simulink model "bpsk_rx_coarse_sync"  (R2020a)
settings: Solver=VariableStepAuto  StartTime=0.0  StopTime=10.0  RelTol=1e-3
undefined symbols (not defined in the file): AXI4, designMultirateFIR, Lite, tx_data, xlfda_numerator
libraries: xbsIndex_r4 x68, hdlsllib x11, dspmlti4 x10, dspswit3 x4, dspsigops x2, commrandsrc3 x1, simulink x1
(part 2 of 2)

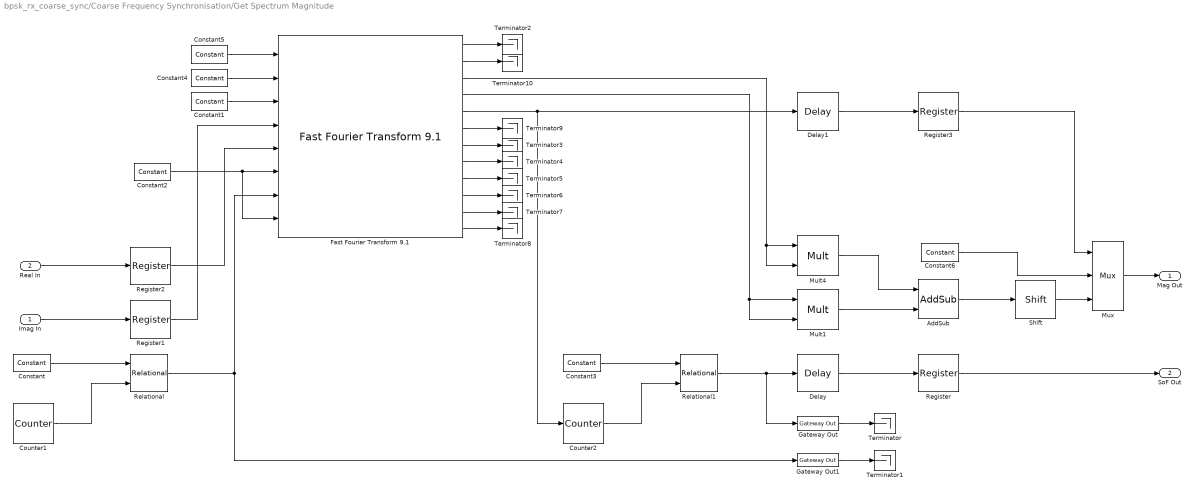
== system bpsk_rx_coarse_sync/Coarse Frequency Synchronisation/Get Spectrum Magnitude ==
  Imag In : Inport
  Real In : Inport  Port=2
  AddSub : xbsIndex_r4/AddSub  mode=Addition  use_carryin=off  use_carryout=off  en=off  latency=1  precision=Full  arith_type=Unsigned  n_bits=16  bin_pt=14  quantization=Truncate  overflow=Wrap  use_behavioral_HDL=off  hw_selection=Fabric  pipelined=off  dbl_ovrd=off  block_type=addsub
  Constant : xbsIndex_r4/Constant  const=1023  gui_display_data_type=Fixed-point  arith_type=Unsigned  n_bits=10  bin_pt=0  preci_type=Single  exp_width=8  frac_width=24  explicit_period=on  period=1/12.8e6  equ=P=C  opselect=C  inp2=PCIN>>17  opr=+  inp1=P  carry=CIN  dbl_ovrd=off  block_type=constant
  Constant1 : xbsIndex_r4/Constant  const=0  gui_display_data_type=Boolean  arith_type=Boolean  n_bits=16  bin_pt=14  preci_type=Single  exp_width=8  frac_width=24  explicit_period=on  period=1/12.8e6  equ=P=C  opselect=C  inp2=PCIN>>17  opr=+  inp1=P  carry=CIN  dbl_ovrd=off  block_type=constant
  Constant2 : xbsIndex_r4/Constant  const=1  gui_display_data_type=Boolean  arith_type=Boolean  n_bits=16  bin_pt=14  preci_type=Single  exp_width=8  frac_width=24  explicit_period=on  period=1/12.8e6  equ=P=C  opselect=C  inp2=PCIN>>17  opr=+  inp1=P  carry=CIN  dbl_ovrd=off  block_type=constant
  Constant3 : xbsIndex_r4/Constant  const=0  gui_display_data_type=Fixed-point  arith_type=Unsigned  n_bits=10  bin_pt=0  preci_type=Single  exp_width=8  frac_width=24  explicit_period=on  period=1/12.8e6  equ=P=C  opselect=C  inp2=PCIN>>17  opr=+  inp1=P  carry=CIN  dbl_ovrd=off  block_type=constant
  Constant4 : xbsIndex_r4/Constant  const=0  gui_display_data_type=Fixed-point  arith_type=Unsigned  n_bits=1  bin_pt=0  preci_type=Single  exp_width=8  frac_width=24  explicit_period=on  period=1/12.8e6  equ=P=C  opselect=C  inp2=PCIN>>17  opr=+  inp1=P  carry=CIN  dbl_ovrd=off  block_type=constant
  Constant5 : xbsIndex_r4/Constant  const=0  gui_display_data_type=Fixed-point  arith_type=Unsigned  n_bits=10  bin_pt=0  preci_type=Single  exp_width=8  frac_width=24  explicit_period=on  period=1/12.8e6  equ=P=C  opselect=C  inp2=PCIN>>17  opr=+  inp1=P  carry=CIN  dbl_ovrd=off  block_type=constant
  Constant6 : xbsIndex_r4/Constant  const=0  gui_display_data_type=Fixed-point  arith_type=Unsigned  n_bits=32  bin_pt=31  preci_type=Single  exp_width=8  frac_width=24  explicit_period=on  period=1/12.8e6  equ=P=C  opselect=C  inp2=PCIN>>17  opr=+  inp1=P  carry=CIN  dbl_ovrd=off  block_type=constant
  Counter1 : xbsIndex_r4/Counter  cnt_type=Count Limited  cnt_to=1023  operation=Up  start_count=0  cnt_by_val=1  arith_type=Unsigned  n_bits=10  bin_pt=0  load_pin=off  rst=off  en=off  explicit_period=on  period=1/12.8e6  use_behavioral_HDL=off  implementation=Fabric  dbl_ovrd=off  block_type=counter
  Counter2 : xbsIndex_r4/Counter  cnt_type=Count Limited  cnt_to=1023  operation=Up  start_count=0  cnt_by_val=1  arith_type=Unsigned  n_bits=10  bin_pt=0  load_pin=off  rst=off  en=on  explicit_period=on  period=1/12.8e6  use_behavioral_HDL=off  implementation=Fabric  dbl_ovrd=off  block_type=counter
  Delay : xbsIndex_r4/Delay  rst=off  infoeditControl=Selection of Reset will increase slice count due to use of real FFs and instead of SRLs  en=off  latency=3  reg_retiming=off  dbl_ovrd=off  block_type=delay
  Delay1 : xbsIndex_r4/Delay  rst=off  infoeditControl=Selection of Reset will increase slice count due to use of real FFs and instead of SRLs  en=off  latency=3  reg_retiming=off  dbl_ovrd=off  block_type=delay
  "Fast Fourier Transform 9.1 " : xbsIndex_r4/Fast Fourier Transform 9.1   transform_length=1024  target_clock_frequency=128  target_data_throughput=13  implementation_options=pipelined_streaming_io  run_time_configurable_transform_length=off  phase_factor_width=16  scaling_options=scaled  rounding_modes=truncation  aclken=off  aresetn=off  output_ordering=natural_order  cyclic_prefix_insertion=off  throttle_scheme=nonrealtime  xk_index=off  ovflo=off  trim_axipin_name=on  memory_options_data=block_ram  memory_options_phase_factors=block_ram  number_of_stages_using_block_ram_for_data_and_phase_factors=1  memory_options_reorder=block_ram  memory_options_hybrid=off  complex_mult_type=use_mults_resources  butterfly_type=use_luts  simulation_type=hybrid_sim  simulation_model=sysgen:xfftv9_cmodel  data_path_portlist={ 's_axis_data_tdata', 'm_axis_data_tdata', 'm_axis_status_tdata', 'event_fft_overflow' }  channels=1  input_ordering=natural_order  input_width=16  ip_name=Fast Fourier Transform  ip_version=9.1  dsptool_ready=true  ipcore_usecache=true  ipcore_useipmodelcache=true  wrapper_available=true  port_translation_map={ 'aclken' => 'en', 'aresetn' => 'rst'}  data_format=fixed_point  block_type=xfft_v9_1
  Gateway Out : xbsIndex_r4/Gateway Out  inherit_from_input=on  hdl_port=off  rows=1  columns=1  UseAsDAC=off  DACChannel='1'  interface=None  automatic_assignment=on  address_offset=hex2dec('00')  intf_name=''  intf_description=''  timing_constraint=None  locs_specified=off  LOCs={}  io_standard={}  block_type=gatewayout
  Gateway Out1 : xbsIndex_r4/Gateway Out  inherit_from_input=on  hdl_port=off  rows=1  columns=1  UseAsDAC=off  DACChannel='1'  interface=None  automatic_assignment=on  address_offset=hex2dec('00')  intf_name=''  intf_description=''  timing_constraint=None  locs_specified=off  LOCs={}  io_standard={}  block_type=gatewayout
  Mult1 : xbsIndex_r4/Mult  precision=User Defined  arith_type=Unsigned  n_bits=63  bin_pt=62  quantization=Truncate  overflow=Saturate  en=off  latency=3  use_behavioral_HDL=off  opt=Speed  use_embedded=on  optimum_pipeline=off  pipeline=on  dbl_ovrd=off  use_rpm=on  placement_style=Triangular  block_type=mult
  Mult4 : xbsIndex_r4/Mult  precision=User Defined  arith_type=Unsigned  n_bits=63  bin_pt=62  quantization=Truncate  overflow=Saturate  en=off  latency=3  use_behavioral_HDL=off  opt=Speed  use_embedded=on  optimum_pipeline=off  pipeline=on  dbl_ovrd=off  use_rpm=on  placement_style=Triangular  block_type=mult
  Mux : xbsIndex_r4/Mux  inputs=2  en=off  latency=0  precision=Full  arith_type=Unsigned  n_bits=16  bin_pt=14  quantization=Truncate  overflow=Wrap  dbl_ovrd=off  block_type=mux
  Register{,1..3} (4 alike) : xbsIndex_r4/Register  init=0  rst=off  en=off  dbl_ovrd=off  block_type=register
  Relational : xbsIndex_r4/Relational  mode=a=b  op_type=Bool  en=off  latency=0  dbl_ovrd=off  block_type=relational
  Relational1 : xbsIndex_r4/Relational  mode=a=b  op_type=Bool  en=off  latency=0  dbl_ovrd=off  block_type=relational
  Shift : xbsIndex_r4/Shift  shift_dir=Right  shift_bits=2  en=off  latency=0  precision=User Defined  arith_type=Unsigned  n_bits=32  bin_pt=31  quantization=Truncate  overflow=Wrap  dbl_ovrd=off  block_type=shift
  Terminator{,1..10} (11 alike) : Terminator
  Mag Out : Outport  VectorParamsAs1DForOutWhenUnconnected=off
  SoF Out : Outport  Port=2  VectorParamsAs1DForOutWhenUnconnected=off
  wires:
  AddSub/1 -> Shift/1
  Mult4/1 -> AddSub/1
  Mult1/1 -> AddSub/2
  Register2/1 -> "Fast Fourier Transform 9.1 "/5
  Register1/1 -> "Fast Fourier Transform 9.1 "/4
  Register/1 -> SoF Out/1
  Delay/1 -> Register/1
  Imag In/1 -> Register1/1
  "Fast Fourier Transform 9.1 "/3 -> Mult4/2, Mult4/1
  Real In/1 -> Register2/1
  "Fast Fourier Transform 9.1 "/4 -> Mult1/1, Mult1/2
  Relational1/1 -> Gateway Out/1, Delay/1
  Constant/1 -> Relational/1
  Relational/1 -> "Fast Fourier Transform 9.1 "/7, Gateway Out1/1
  Gateway Out/1 -> Terminator/1
  Gateway Out1/1 -> Terminator1/1
  Counter1/1 -> Relational/2
  "Fast Fourier Transform 9.1 "/1 -> Terminator2/1
  Constant1/1 -> "Fast Fourier Transform 9.1 "/3
  "Fast Fourier Transform 9.1 "/7 -> Terminator3/1
  "Fast Fourier Transform 9.1 "/8 -> Terminator4/1
  "Fast Fourier Transform 9.1 "/9 -> Terminator5/1
  "Fast Fourier Transform 9.1 "/10 -> Terminator6/1
  "Fast Fourier Transform 9.1 "/11 -> Terminator7/1
  "Fast Fourier Transform 9.1 "/12 -> Terminator8/1
  Constant2/1 -> "Fast Fourier Transform 9.1 "/8, "Fast Fourier Transform 9.1 "/6
  Counter2/1 -> Relational1/2
  Constant3/1 -> Relational1/1
  "Fast Fourier Transform 9.1 "/5 -> Delay1/1, Counter2/1
  "Fast Fourier Transform 9.1 "/6 -> Terminator9/1
  Constant4/1 -> "Fast Fourier Transform 9.1 "/2
  Constant5/1 -> "Fast Fourier Transform 9.1 "/1
  "Fast Fourier Transform 9.1 "/2 -> Terminator10/1
  Mux/1 -> Mag Out/1
  Shift/1 -> Mux/3
  Constant6/1 -> Mux/2
  Delay1/1 -> Register3/1
  Register3/1 -> Mux/1

== system bpsk_rx_coarse_sync/Coarse Frequency Synchronisation/Increase Signal Power ==
  note: Product block is required as it is a complex multiplication
  note: 18-bit multiply for DSP48E2
  Imag In : Inport
  Real In : Inport  Port=2
  Convert : xbsIndex_r4/Convert  gui_display_data_type=Fixed-point  arith_type="Signed  (2's comp)"  n_bits=32  bin_pt=31  float_type=Single  exp_bits=8  fraction_bits=24  quantization=Truncate  overflow=Wrap  en=off  latency=0  pipeline=off  dbl_ovrd=off  block_type=convert
  Convert1 : xbsIndex_r4/Convert  gui_display_data_type=Fixed-point  arith_type="Signed  (2's comp)"  n_bits=32  bin_pt=31  float_type=Single  exp_bits=8  fraction_bits=24  quantization=Truncate  overflow=Wrap  en=off  latency=0  pipeline=off  dbl_ovrd=off  block_type=convert
  Convert2 : xbsIndex_r4/Convert  gui_display_data_type=Fixed-point  arith_type="Signed  (2's comp)"  n_bits=18  bin_pt=15  float_type=Single  exp_bits=8  fraction_bits=24  quantization=Truncate  overflow=Wrap  en=off  latency=0  pipeline=off  dbl_ovrd=off  block_type=convert
  Convert4 : xbsIndex_r4/Convert  gui_display_data_type=Fixed-point  arith_type="Signed  (2's comp)"  n_bits=18  bin_pt=15  float_type=Single  exp_bits=8  fraction_bits=24  quantization=Truncate  overflow=Wrap  en=off  latency=0  pipeline=off  dbl_ovrd=off  block_type=convert
  Product1 : xbsIndex_r4/Product  complex_multiplier=on  optimizegoal=Performance  simulation_type=fast_sim  simulation_model=sysgen:product_macro  block_type=product_macro
  Product2 : xbsIndex_r4/Product  complex_multiplier=on  optimizegoal=Performance  simulation_type=fast_sim  simulation_model=sysgen:product_macro  block_type=product_macro
  Imag Out : Outport  VectorParamsAs1DForOutWhenUnconnected=off
  Real Out : Outport  Port=2  VectorParamsAs1DForOutWhenUnconnected=off
  wires:
  Convert1/1 -> Imag Out/1
  Convert/1 -> Real Out/1
  Product1/2 -> Convert1/1
  Product1/1 -> Convert/1
  Convert2/1 -> Product1/2, Product1/4
  Convert4/1 -> Product1/3, Product1/1
  Product2/2 -> Convert2/1
  Product2/1 -> Convert4/1
  Real In/1 -> Product2/3, Product2/1
  Imag In/1 -> Product2/4, Product2/2

== system bpsk_rx_coarse_sync/Coarse Frequency Synchronisation/NCO ==
  Offset In : Inport
  AddSub : xbsIndex_r4/AddSub  mode=Addition  use_carryin=off  use_carryout=off  en=off  latency=0  precision=User Defined  arith_type=Unsigned  n_bits=41  bin_pt=41-10  quantization=Truncate  overflow=Wrap  use_behavioral_HDL=off  hw_selection=Fabric  pipelined=off  dbl_ovrd=off  block_type=addsub
  CMult : xbsIndex_r4/CMult  const=1024/(12.8e6)  gui_display_data_type=Fixed-point  const_n_bits=i+b  const_bin_pt=b  float_type=Single  exp_bits=8  fraction_bits=24  en=off  latency=1  precision=User Defined  arith_type="Signed  (2's comp)"  n_bits=n+b  bin_pt=b  quantization=Truncate  overflow=Saturate  use_behavioral_HDL=off  mem_type=Distributed RAM  pipeline=off  dbl_ovrd=off  block_type=cmult
  Convert4 : xbsIndex_r4/Convert  gui_display_data_type=Fixed-point  arith_type=Unsigned  n_bits=10  bin_pt=0  float_type=Single  exp_bits=8  fraction_bits=24  quantization=Truncate  overflow=Wrap  en=off  latency=0  pipeline=off  dbl_ovrd=off  block_type=convert
  Delay2 : xbsIndex_r4/Delay  rst=off  infoeditControl=Selection of Reset will increase slice count due to use of real FFs and instead of SRLs  en=off  latency=1  reg_retiming=off  dbl_ovrd=off  block_type=delay
  Sin_ROM : xbsIndex_r4/ROM  depth=1024  initVector=sin(pi*(0:1024-1)/(1024/2))  distributed_mem=Block RAM  rst=off  init_reg=0  en=off  latency=1  gui_display_data_type=Fixed-point  arith_type="Signed  (2's comp)"  n_bits=L  bin_pt=L-2  preci_type=Single  exp_width=8  frac_width=24  optimize=Area  use_rpm=on  dbl_ovrd=off  simulation_type=fast_sim  block_type=sprom
  cos_ROM : xbsIndex_r4/ROM  depth=1024  initVector=cos(pi*(0:1024-1)/(1024/2))  distributed_mem=Block RAM  rst=off  init_reg=0  en=off  latency=1  gui_display_data_type=Fixed-point  arith_type="Signed  (2's comp)"  n_bits=L  bin_pt=L-2  preci_type=Single  exp_width=8  frac_width=24  optimize=Area  use_rpm=on  dbl_ovrd=off  simulation_type=fast_sim  block_type=sprom
  cos : Outport  VectorParamsAs1DForOutWhenUnconnected=off
  sin : Outport  Port=2  VectorParamsAs1DForOutWhenUnconnected=off
  wires:
  AddSub/1 -> Convert4/1, Delay2/1
  Offset In/1 -> CMult/1
  Delay2/1 -> AddSub/1
  CMult/1 -> AddSub/2
  Convert4/1 -> Sin_ROM/1, cos_ROM/1
  Sin_ROM/1 -> sin/1
  cos_ROM/1 -> cos/1

== system bpsk_rx_coarse_sync/BPSK System/BPSK TX Generation/DBPSK Modulator ==
  Input : Inport
  Cast To Boolean : DataTypeConversion  OutDataTypeStr=boolean
  Constant : Constant  Value=fi(1, 1, 16, 14)  OutDataTypeStr=fixdt(1,16,14)  SampleTime=-1
  Constant1 : Constant  Value=fi(-1, 1, 16, 14)  OutDataTypeStr=fixdt(1,16,14)  SampleTime=-1
  Constant2 : Constant  Value=0  OutDataTypeStr=Inherit: Inherit via back propagation  SampleTime=-1
  Delay : Delay  DelayLength=1
  Multiport Switch : MultiPortSwitch  DataPortOrder=Zero-based contiguous  Inputs=2  zeroidx=on
  Real-Imag to Complex : RealImagToComplex
  XOR : Logic  Operator=XOR  IconShape=distinctive  AllPortsSameDT=off  OutDataTypeStr=boolean
  Output : Outport  VectorParamsAs1DForOutWhenUnconnected=off
  wires:
  Constant2/1 -> Real-Imag to Complex/2
  Real-Imag to Complex/1 -> Output/1
  Multiport Switch/1 -> Real-Imag to Complex/1
  Constant1/1 -> Multiport Switch/3
  Constant/1 -> Multiport Switch/2
  Input/1 -> Cast To Boolean/1
  Delay/1 -> XOR/1
  XOR/1 -> Multiport Switch/1, Delay/1
  Cast To Boolean/1 -> XOR/2

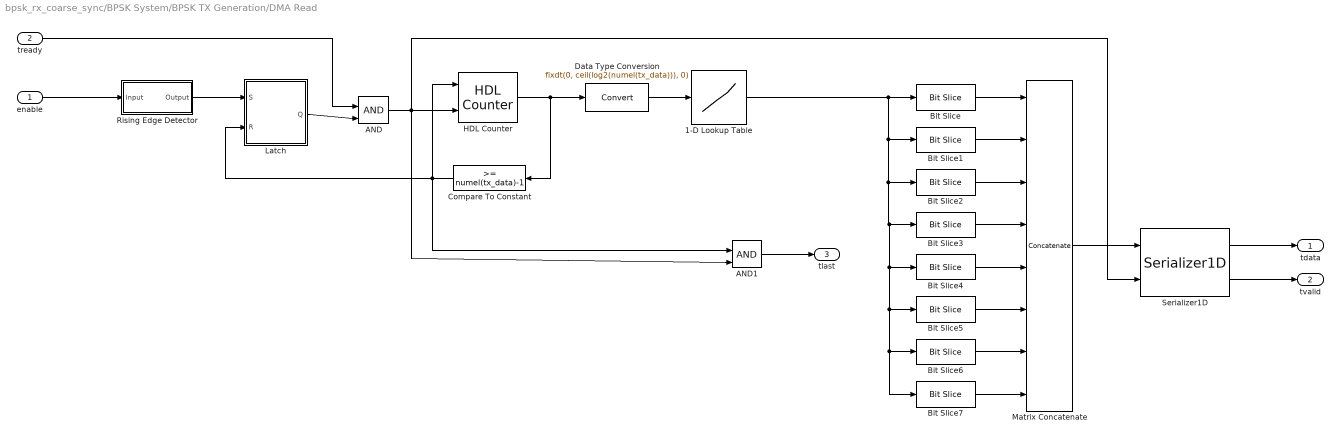
== system bpsk_rx_coarse_sync/BPSK System/BPSK TX Generation/DMA Read ==
  enable : Inport
  tready : Inport  Port=2
  1-D Lookup Table : Lookup_n-D  NumberOfTableDimensions=1  BreakpointsForDimension1=[0:1:numel(tx_data)-1]  Table=tx_data  TableDataTypeStr=Inherit: Inherit from 'Table data'  ExtrapMethod=Clip  InternalRulePriority=Speed  OutDataTypeStr=Inherit: Inherit from 'Table data'  RndMeth=Simplest  InputSameDT=on
  AND : Logic  IconShape=distinctive  AllPortsSameDT=off  OutDataTypeStr=boolean
  AND1 : Logic  IconShape=distinctive  AllPortsSameDT=off  OutDataTypeStr=boolean
  Bit Slice : hdlsllib/Logic and Bit Operations/Bit Slice  lidx=0  ridx=0
      settings: SourceProductBaseCode=SL
  Bit Slice1 : hdlsllib/Logic and Bit Operations/Bit Slice  lidx=1  ridx=1
      settings: SourceProductBaseCode=SL
  Bit Slice2 : hdlsllib/Logic and Bit Operations/Bit Slice  lidx=2  ridx=2
      settings: SourceProductBaseCode=SL
  Bit Slice3 : hdlsllib/Logic and Bit Operations/Bit Slice  lidx=3  ridx=3
      settings: SourceProductBaseCode=SL
  Bit Slice4 : hdlsllib/Logic and Bit Operations/Bit Slice  lidx=4  ridx=4
      settings: SourceProductBaseCode=SL
  Bit Slice5 : hdlsllib/Logic and Bit Operations/Bit Slice  lidx=5  ridx=5
      settings: SourceProductBaseCode=SL
  Bit Slice6 : hdlsllib/Logic and Bit Operations/Bit Slice  lidx=6  ridx=6
      settings: SourceProductBaseCode=SL
  Bit Slice7 : hdlsllib/Logic and Bit Operations/Bit Slice  lidx=7  ridx=7
      settings: SourceProductBaseCode=SL
  Compare To Constant : simulink/Logic and Bit Operations/Compare To Constant  relop=>=  const=numel(tx_data)-1  OutDataTypeStr=boolean
  Data Type Conversion : DataTypeConversion  OutDataTypeStr=fixdt(0, ceil(log2(numel(tx_data))), 0)
  HDL Counter : hdlsllib/Sources/HDL Counter  CountType=Free running  CountInit=0  CountStep=1  CountMax=25  CountFromType=Initial value  CountFrom=0  CountResetPort=on  CountLoadPort=off  CountEnbPort=on  CountDirPort=off  CountDataType=Unsigned  CountWordLen=32  CountFracLen=0  CountSampTime=1
  Latch : Subsystem
  Matrix Concatenate : Concatenate  NumInputs=8  Mode=Multidimensional array  ConcatenateDimension=2
  Rising Edge Detector : Subsystem
  Serializer1D : hdlsllib/HDL Operations/Serializer1D  Ratio=8  IdleCycles=0  validIn=on  startOut=off  validOut=on  inputDataDimensions=-1  inputSampleTime=-1  inputSignalType=auto
      settings: SourceProductBaseCode=SL
  tdata : Outport  VectorParamsAs1DForOutWhenUnconnected=off
  tvalid : Outport  Port=2  VectorParamsAs1DForOutWhenUnconnected=off
  tlast : Outport  Port=3  VectorParamsAs1DForOutWhenUnconnected=off
  wires:
  Serializer1D/2 -> tvalid/1
  Bit Slice5/1 -> Matrix Concatenate/6
  Bit Slice6/1 -> Matrix Concatenate/7
  Bit Slice7/1 -> Matrix Concatenate/8
  Bit Slice4/1 -> Matrix Concatenate/5
  Serializer1D/1 -> tdata/1
  1-D Lookup Table/1 -> Bit Slice/1, Bit Slice1/1, Bit Slice2/1, Bit Slice3/1, Bit Slice4/1, Bit Slice5/1, Bit Slice6/1, Bit Slice7/1
  Bit Slice2/1 -> Matrix Concatenate/3
  Bit Slice1/1 -> Matrix Concatenate/2
  Bit Slice3/1 -> Matrix Concatenate/4
  Bit Slice/1 -> Matrix Concatenate/1
  Matrix Concatenate/1 -> Serializer1D/1
  Compare To Constant/1 -> AND1/1, HDL Counter/1, Latch/2(R)
  enable/1 -> Rising Edge Detector/1(Input)
  HDL Counter/1 -> Compare To Constant/1, Data Type Conversion/1
  Data Type Conversion/1 -> 1-D Lookup Table/1
  Rising Edge Detector/1(Output) -> Latch/1(S)
  AND/1 -> AND1/2, Serializer1D/2, HDL Counter/2
  Latch/1(Q) -> AND/2
  tready/1 -> AND/1
  AND1/1 -> tlast/1

== system bpsk_rx_coarse_sync/BPSK System/RF-ADC/Decimation Filter ==
  Data In : Inport
  FIR 0 : dspmlti4/FIR Decimation  FilterSource=Filter object  h=designMultirateFIR(1,2)  D=2  filtStruct=Direct form  FilterObject=fir0  InputProcessing=Columns as channels (frame based)  framing=Allow multirate processing  inputOffset=0  outputBufInitCond=0  roundingMode=Floor  overflowMode=off  firstCoeffDataTypeStr=Inherit: Same word length as input  firstCoeffMin=[]  firstCoeffMax=[]  firstCoeffLastDataTypeStr=Inherit: Same word length as input  outputDataTypeStr=Inherit: Same as accumulator  outputMin=[]  outputMax=[]  outputLastDataTypeStr=Inherit: Same as accumulator
  FIR 1 : dspmlti4/FIR Decimation  FilterSource=Filter object  h=designMultirateFIR(1,2)  D=2  filtStruct=Direct form  FilterObject=fir1  InputProcessing=Columns as channels (frame based)  framing=Allow multirate processing  inputOffset=0  outputBufInitCond=0  roundingMode=Floor  overflowMode=off  firstCoeffDataTypeStr=Inherit: Same word length as input  firstCoeffMin=[]  firstCoeffMax=[]  firstCoeffLastDataTypeStr=Inherit: Same word length as input  outputDataTypeStr=Inherit: Same as accumulator  outputMin=[]  outputMax=[]  outputLastDataTypeStr=Inherit: Same as accumulator
  FIR 2 : dspmlti4/FIR Decimation  FilterSource=Filter object  h=designMultirateFIR(1,2)  D=2  filtStruct=Direct form  FilterObject=fir2  InputProcessing=Columns as channels (frame based)  framing=Allow multirate processing  inputOffset=0  outputBufInitCond=0  roundingMode=Floor  overflowMode=off  firstCoeffDataTypeStr=Inherit: Same word length as input  firstCoeffMin=[]  firstCoeffMax=[]  firstCoeffLastDataTypeStr=Inherit: Same word length as input  outputDataTypeStr=Inherit: Same as accumulator  outputMin=[]  outputMax=[]  outputLastDataTypeStr=Inherit: Same as accumulator
  Data Out : Outport  VectorParamsAs1DForOutWhenUnconnected=off
  wires:
  FIR 2/1 -> FIR 1/1
  Data In/1 -> FIR 2/1
  FIR 0/1 -> Data Out/1
  FIR 1/1 -> FIR 0/1

== system bpsk_rx_coarse_sync/BPSK System/RF-ADC/NCO and Mixer ==
  Data In : Inport
  Constant1 : Constant  Value=m  OutDataTypeStr=fixdt(0,2,0)  SampleTime=-1
  Data Type Conversion : DataTypeConversion  OutDataTypeStr=fixdt(1,16,14)
  Multiport Switch1 : MultiPortSwitch  DataPortOrder=Zero-based contiguous  zeroidx=on
  RF-ADC Coarse Mixer : Subsystem
  RF-ADC Fine Mixer : Subsystem
  Real-Imag to Complex : RealImagToComplex
  Data Out : Outport  VectorParamsAs1DForOutWhenUnconnected=off
  wires:
  Data Type Conversion/1 -> Multiport Switch1/2
  Constant1/1 -> Multiport Switch1/1
  Data In/1 -> Real-Imag to Complex/2, RF-ADC Fine Mixer/1(Data In), RF-ADC Coarse Mixer/1(Data In), Real-Imag to Complex/1
  RF-ADC Coarse Mixer/1(Data Out) -> Multiport Switch1/3
  Real-Imag to Complex/1 -> Data Type Conversion/1
  RF-ADC Fine Mixer/1(Data Out) -> Multiport Switch1/4
  Multiport Switch1/1 -> Data Out/1

== system bpsk_rx_coarse_sync/BPSK System/RF-ADC/RF-ADC ==
  Data In : Inport
  Buffer : Buffer  N=ssr  OutputFrames=off
  Data Type Conversion : DataTypeConversion  OutDataTypeStr=fixdt(1,12,10)
  Rate Transition : RateTransition  OutPortSampleTime=1/fs
  Data Out : Outport  VectorParamsAs1DForOutWhenUnconnected=off
  wires:
  Buffer/1 -> Data Out/1
  Data Type Conversion/1 -> Buffer/1
  Data In/1 -> Rate Transition/1
  Rate Transition/1 -> Data Type Conversion/1

== system bpsk_rx_coarse_sync/BPSK System/RF-DAC/Coarse Delay ==
  Data In : Inport
  Data Out : Outport  VectorParamsAs1DForOutWhenUnconnected=off
  wires:
  Data In/1 -> Data Out/1

== system bpsk_rx_coarse_sync/BPSK System/RF-DAC/Interpolation Filter ==
  Data In : Inport
  FIR 0 : dspmlti4/FIR Interpolation  FilterSource=Filter object  PrivateCoeffs=0  h=designMultirateFIR(3,1)  L=2  FilterObject=fir0  InputProcessing=Columns as channels (frame based)  framing=Allow multirate processing  outputBufInitCond=0  roundingMode=Floor  overflowMode=off  firstCoeffDataTypeStr=Inherit: Same word length as input  firstCoeffMin=[]  firstCoeffMax=[]  firstCoeffLastDataTypeStr=Inherit: Same word length as input  outputDataTypeStr=Inherit: Same as accumulator  outputMin=[]  outputMax=[]  outputLastDataTypeStr=Inherit: Same as accumulator
  FIR 1 : dspmlti4/FIR Interpolation  FilterSource=Filter object  PrivateCoeffs=0  h=designMultirateFIR(3,1)  L=2  FilterObject=fir1  InputProcessing=Columns as channels (frame based)  framing=Allow multirate processing  outputBufInitCond=0  roundingMode=Floor  overflowMode=off  firstCoeffDataTypeStr=Inherit: Same word length as input  firstCoeffMin=[]  firstCoeffMax=[]  firstCoeffLastDataTypeStr=Inherit: Same word length as input  outputDataTypeStr=Inherit: Same as accumulator  outputMin=[]  outputMax=[]  outputLastDataTypeStr=Inherit: Same as accumulator
  FIR 2 : dspmlti4/FIR Interpolation  FilterSource=Filter object  PrivateCoeffs=0  h=designMultirateFIR(3,1)  L=2  FilterObject=fir2  InputProcessing=Columns as channels (frame based)  framing=Allow multirate processing  outputBufInitCond=0  roundingMode=Floor  overflowMode=off  firstCoeffDataTypeStr=Inherit: Same word length as input  firstCoeffMin=[]  firstCoeffMax=[]  firstCoeffLastDataTypeStr=Inherit: Same word length as input  outputDataTypeStr=Inherit: Same as accumulator  outputMin=[]  outputMax=[]  outputLastDataTypeStr=Inherit: Same as accumulator
  Data Out : Outport  VectorParamsAs1DForOutWhenUnconnected=off
  wires:
  FIR 1/1 -> FIR 0/1
  FIR 0/1 -> Data Out/1
  Data In/1 -> FIR 2/1
  FIR 2/1 -> FIR 1/1

== system bpsk_rx_coarse_sync/BPSK System/RF-DAC/NCO and Mixer ==
  Data In : Inport
  Complex to Real-Imag : ComplexToRealImag
  Constant1 : Constant  Value=m  OutDataTypeStr=fixdt(0,2,0)  SampleTime=-1
  Multiport Switch1 : MultiPortSwitch  DataPortOrder=Zero-based contiguous  zeroidx=on
  RF-DAC Coarse Mixer : Subsystem
  RF-DAC Fine Mixer : Subsystem
  Terminator : Terminator
  Data Out : Outport  VectorParamsAs1DForOutWhenUnconnected=off
  wires:
  Complex to Real-Imag/2 -> Terminator/1
  Complex to Real-Imag/1 -> Multiport Switch1/2
  RF-DAC Fine Mixer/1(Data Out) -> Multiport Switch1/4
  Multiport Switch1/1 -> Data Out/1
  Data In/1 -> RF-DAC Fine Mixer/1(Data In), RF-DAC Coarse Mixer/1(Data In), Complex to Real-Imag/1
  Constant1/1 -> Multiport Switch1/1
  RF-DAC Coarse Mixer/1(Data Out) -> Multiport Switch1/3

== system bpsk_rx_coarse_sync/BPSK System/RF-DAC/Output Filter ==
  Data In : Inport
  Data Out : Outport  VectorParamsAs1DForOutWhenUnconnected=off
  wires:
  Data In/1 -> Data Out/1

== system bpsk_rx_coarse_sync/BPSK System/RF-DAC/QMC Gain & Phase ==
  Data In : Inport
  Data Out : Outport  VectorParamsAs1DForOutWhenUnconnected=off
  wires:
  Data In/1 -> Data Out/1

== system bpsk_rx_coarse_sync/BPSK System/RF-DAC/QMC Threshold ==
  Data In : Inport
  Data Out : Outport  VectorParamsAs1DForOutWhenUnconnected=off
  wires:
  Data In/1 -> Data Out/1

== system bpsk_rx_coarse_sync/BPSK System/RF-DAC/RF-DAC ==
  Data In : Inport
  Cast To Double : DataTypeConversion  OutDataTypeStr=double
  Rate Transition : RateTransition  OutPortSampleTime=0
  Unbuffer : Unbuffer
  Data Out : Outport  VectorParamsAs1DForOutWhenUnconnected=off
  wires:
  Rate Transition/1 -> Data Out/1
  Data In/1 -> Unbuffer/1
  Unbuffer/1 -> Cast To Double/1
  Cast To Double/1 -> Rate Transition/1

== system bpsk_rx_coarse_sync/BPSK System/BPSK TX Generation/DMA Read/Latch ==
  S : Inport
  R : Inport  Port=2
  Multiport Switch : MultiPortSwitch  DataPortOrder=Zero-based contiguous  Inputs=2  zeroidx=on
  Unit Delay Resettable Synchronous : hdlsllib/Discrete/Unit Delay Resettable Synchronous  InitialCondition=0.0  SampleTime=-1
      settings: SourceProductBaseCode=SL
  Q : Outport  VectorParamsAs1DForOutWhenUnconnected=off
  wires:
  Multiport Switch/1 -> Unit Delay Resettable Synchronous/1, Q/1
  S/1 -> Multiport Switch/3, Multiport Switch/1
  Unit Delay Resettable Synchronous/1 -> Multiport Switch/2
  R/1 -> Unit Delay Resettable Synchronous/2

== system bpsk_rx_coarse_sync/BPSK System/BPSK TX Generation/DMA Read/Rising Edge Detector ==
  Input : Inport
  AND1 : Logic  IconShape=distinctive  AllPortsSameDT=off  OutDataTypeStr=boolean
  Delay1 : Delay  DelayLength=1
  NOT : Logic  Operator=NOT  IconShape=distinctive  AllPortsSameDT=off  OutDataTypeStr=boolean
  Output : Outport  VectorParamsAs1DForOutWhenUnconnected=off
  wires:
  NOT/1 -> AND1/1
  Input/1 -> AND1/2, Delay1/1
  Delay1/1 -> NOT/1
  AND1/1 -> Output/1

== system bpsk_rx_coarse_sync/BPSK System/RF-ADC/NCO and Mixer/RF-ADC Coarse Mixer ==
  Data In : Inport
  Constant : Constant  Value=mc  OutDataTypeStr=fixdt(0,2,0)  SampleTime=-1
  Data Type Conversion : DataTypeConversion  OutDataTypeStr=fixdt(1,16,14)
  Multiport Switch1 : MultiPortSwitch  DataPortOrder=Zero-based contiguous  zeroidx=on
  Negate : Subsystem
  fs_2 : Subsystem
  fs_4 : Subsystem
  Data Out : Outport  VectorParamsAs1DForOutWhenUnconnected=off
  wires:
  Data Type Conversion/1 -> Data Out/1
  fs_4/1(Data Out) -> Multiport Switch1/3, Negate/1(Data In)
  Negate/1(Data Out) -> Multiport Switch1/4
  Data In/1 -> fs_2/1(Data In), fs_4/1(Data In)
  Constant/1 -> Multiport Switch1/1
  fs_2/1(Data Out) -> Multiport Switch1/2
  Multiport Switch1/1 -> Data Type Conversion/1

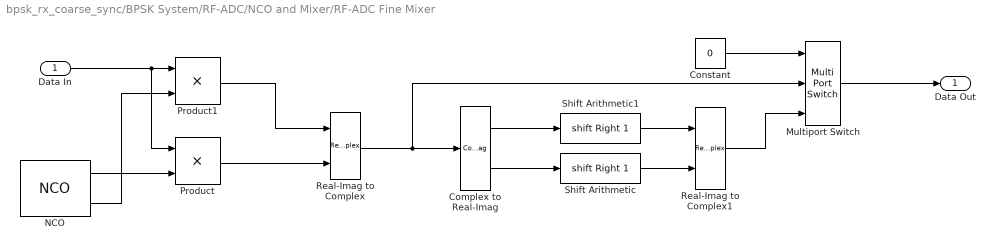
== system bpsk_rx_coarse_sync/BPSK System/RF-ADC/NCO and Mixer/RF-ADC Fine Mixer ==
  Data In : Inport
  Complex to Real-Imag : ComplexToRealImag
  Constant : Constant  Value=0  SampleTime=-1
  Multiport Switch : MultiPortSwitch  DataPortOrder=Zero-based contiguous  Inputs=2  zeroidx=on
  NCO : dspsigops/NCO  AccIncSrc=Specify via dialog  AccInc=fix((((fc*1e9)*(2^18))/(fs))*2^30)  PhaseOffsetSrc=Specify via dialog  PhaseOffset=fix((((2^18)*fph)/(2*pi))*2^30)  AccumWL=48  HasDither=off  DitherWL=4  PNgeneratorLength=19  HasPhaseQuantizer=on  TableDepth=18  HasOutputPhaseError=off  Formula=Sine and cosine  DataType=Binary point scaling  OutputWL=16  OutputFL=14  CompMethod=Table lookup (no interpolation)  SampleTime=1/(fs)  SamplesPerFrame=ssr  OutputFrames=off
      settings: SourceProductBaseCode=DS
  Product : Product  OutDataTypeStr=fixdt(1,16,14)
  Product1 : Product  OutDataTypeStr=fixdt(1,16,14)
  Real-Imag to Complex : RealImagToComplex
  Real-Imag to Complex1 : RealImagToComplex
  Shift Arithmetic : ArithShift  BitShiftNumber=1  BitShiftDirection=Right
  Shift Arithmetic1 : ArithShift  BitShiftNumber=1  BitShiftDirection=Right
  Data Out : Outport  VectorParamsAs1DForOutWhenUnconnected=off
  wires:
  Product/1 -> Real-Imag to Complex/2
  Product1/1 -> Real-Imag to Complex/1
  Real-Imag to Complex/1 -> Complex to Real-Imag/1, Multiport Switch/2
  NCO/2 -> Product1/2
  NCO/1 -> Product/2
  Real-Imag to Complex1/1 -> Multiport Switch/3
  Shift Arithmetic/1 -> Real-Imag to Complex1/2
  Shift Arithmetic1/1 -> Real-Imag to Complex1/1
  Complex to Real-Imag/1 -> Shift Arithmetic1/1
  Complex to Real-Imag/2 -> Shift Arithmetic/1
  Multiport Switch/1 -> Data Out/1
  Constant/1 -> Multiport Switch/1
  Data In/1 -> Product/1, Product1/1

== system bpsk_rx_coarse_sync/BPSK System/RF-DAC/NCO and Mixer/RF-DAC Coarse Mixer ==
  Data In : Inport
  Add2 : Sum
  Complex to Real-Imag : ComplexToRealImag
  Constant : Constant  Value=mc  OutDataTypeStr=fixdt(0,2,0)  SampleTime=-1
  Multiport Switch1 : MultiPortSwitch  DataPortOrder=Zero-based contiguous  zeroidx=on
  Negate : Subsystem
  fs_2 : Subsystem
  fs_4 : Subsystem
  Data Out : Outport  VectorParamsAs1DForOutWhenUnconnected=off
  wires:
  Add2/1 -> Data Out/1
  Complex to Real-Imag/2 -> Add2/2
  Complex to Real-Imag/1 -> Add2/1
  Multiport Switch1/1 -> Complex to Real-Imag/1
  fs_2/1(Data Out) -> Multiport Switch1/2
  Constant/1 -> Multiport Switch1/1
  Data In/1 -> fs_4/1(Data In), fs_2/1(Data In)
  Negate/1(Data Out) -> Multiport Switch1/4
  fs_4/1(Data Out) -> Negate/1(Data In), Multiport Switch1/3

== system bpsk_rx_coarse_sync/BPSK System/RF-DAC/NCO and Mixer/RF-DAC Fine Mixer ==
  Data In : Inport
  Add2 : Sum
  Complex to Real-Imag1 : ComplexToRealImag
  Constant : Constant  Value=0  OutDataTypeStr=boolean  SampleTime=-1
  Multiport Switch : MultiPortSwitch  DataPortOrder=Zero-based contiguous  Inputs=2  zeroidx=on
  NCO : dspsigops/NCO  AccIncSrc=Specify via dialog  AccInc=fix((((fc*1e9)*(2^18))/(fs))*2^30)  PhaseOffsetSrc=Specify via dialog  PhaseOffset=fix((((2^18)*fph)/(2*pi))*2^30)  AccumWL=48  HasDither=off  DitherWL=4  PNgeneratorLength=19  HasPhaseQuantizer=on  TableDepth=18  HasOutputPhaseError=off  Formula=Sine and cosine  DataType=Binary point scaling  OutputWL=16  OutputFL=14  CompMethod=Table lookup (no interpolation)  SampleTime=1/(fs)  SamplesPerFrame=ssr  OutputFrames=off
      settings: SourceProductBaseCode=DS
  Product1 : Product  OutDataTypeStr=Inherit: Same as first input
  Product4 : Product  OutDataTypeStr=Inherit: Same as first input
  Shift Arithmetic1 : ArithShift  BitShiftNumber=1  BitShiftDirection=Right
  Data Out : Outport  VectorParamsAs1DForOutWhenUnconnected=off
  wires:
  Product1/1 -> Add2/2
  Complex to Real-Imag1/2 -> Product4/1
  Complex to Real-Imag1/1 -> Product1/2
  NCO/2 -> Product1/1
  NCO/1 -> Product4/2
  Product4/1 -> Add2/1
  Data In/1 -> Complex to Real-Imag1/1
  Constant/1 -> Multiport Switch/1
  Multiport Switch/1 -> Data Out/1
  Add2/1 -> Shift Arithmetic1/1, Multiport Switch/2
  Shift Arithmetic1/1 -> Multiport Switch/3

== system bpsk_rx_coarse_sync/BPSK System/RF-ADC/NCO and Mixer/RF-ADC Coarse Mixer/Negate ==
  Data In : Inport
  Complex to Real-Imag2 : ComplexToRealImag
  Real-Imag to Complex1 : RealImagToComplex
  Unary Minus : UnaryMinus
  Data Out : Outport  VectorParamsAs1DForOutWhenUnconnected=off
  wires:
  Complex to Real-Imag2/1 -> Real-Imag to Complex1/1
  Real-Imag to Complex1/1 -> Data Out/1
  Data In/1 -> Complex to Real-Imag2/1
  Unary Minus/1 -> Real-Imag to Complex1/2
  Complex to Real-Imag2/2 -> Unary Minus/1

== system bpsk_rx_coarse_sync/BPSK System/RF-ADC/NCO and Mixer/RF-ADC Coarse Mixer/fs_2 ==
  Data In : Inport
  Counter : dspswit3/Counter  Direction=Up  CountEvent=Free running  CounterSize=User defined  MaxCount=1  InitialCount=0  Output=Count  HitValue=32  ResetInput=off  SamplesPerFrame=ssr  Ts=1/(fs)  CntDtype=uint8  HitDtype=Logical
  Multiport Switch2 : MultiPortSwitch  DataPortOrder=Zero-based contiguous  Inputs=2  zeroidx=on
  Real-Imag to Complex : RealImagToComplex
  Real-Imag to Complex1 : RealImagToComplex
  Unary Minus1 : UnaryMinus
  Data Out : Outport  VectorParamsAs1DForOutWhenUnconnected=off
  wires:
  Unary Minus1/1 -> Real-Imag to Complex/1, Real-Imag to Complex/2
  Counter/1 -> Multiport Switch2/1
  Multiport Switch2/1 -> Data Out/1
  Real-Imag to Complex/1 -> Multiport Switch2/3
  Real-Imag to Complex1/1 -> Multiport Switch2/2
  Data In/1 -> Unary Minus1/1, Real-Imag to Complex1/2, Real-Imag to Complex1/1

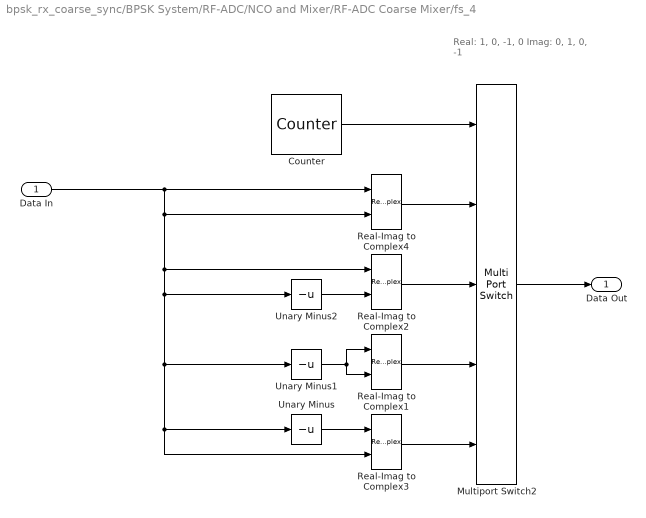
== system bpsk_rx_coarse_sync/BPSK System/RF-ADC/NCO and Mixer/RF-ADC Coarse Mixer/fs_4 ==
  note: Real:	1, 0, -1, 0
      | Imag:	0, 1, 0, -1
  Data In : Inport
  Counter : dspswit3/Counter  Direction=Up  CountEvent=Free running  CounterSize=User defined  MaxCount=3  InitialCount=0  Output=Count  HitValue=32  ResetInput=off  SamplesPerFrame=ssr  Ts=1/(fs)  CntDtype=uint8  HitDtype=Logical
  Multiport Switch2 : MultiPortSwitch  DataPortOrder=Zero-based contiguous  Inputs=4  zeroidx=on
  Real-Imag to Complex{1..4} (4 alike) : RealImagToComplex
  Unary Minus : UnaryMinus
  Unary Minus1 : UnaryMinus
  Unary Minus2 : UnaryMinus
  Data Out : Outport  VectorParamsAs1DForOutWhenUnconnected=off
  wires:
  Multiport Switch2/1 -> Data Out/1
  Real-Imag to Complex3/1 -> Multiport Switch2/5
  Data In/1 -> Real-Imag to Complex4/2, Real-Imag to Complex2/1, Real-Imag to Complex3/2, Unary Minus/1, Unary Minus1/1, Unary Minus2/1, Real-Imag to Complex4/1
  Real-Imag to Complex2/1 -> Multiport Switch2/3
  Counter/1 -> Multiport Switch2/1
  Real-Imag to Complex1/1 -> Multiport Switch2/4
  Unary Minus1/1 -> Real-Imag to Complex1/1, Real-Imag to Complex1/2
  Real-Imag to Complex4/1 -> Multiport Switch2/2
  Unary Minus2/1 -> Real-Imag to Complex2/2
  Unary Minus/1 -> Real-Imag to Complex3/1

== system bpsk_rx_coarse_sync/BPSK System/RF-DAC/NCO and Mixer/RF-DAC Coarse Mixer/Negate ==
  Data In : Inport
  Complex to Real-Imag2 : ComplexToRealImag
  Real-Imag to Complex1 : RealImagToComplex
  Unary Minus : UnaryMinus
  Data Out : Outport  VectorParamsAs1DForOutWhenUnconnected=off
  wires:
  Complex to Real-Imag2/2 -> Unary Minus/1
  Unary Minus/1 -> Real-Imag to Complex1/2
  Data In/1 -> Complex to Real-Imag2/1
  Real-Imag to Complex1/1 -> Data Out/1
  Complex to Real-Imag2/1 -> Real-Imag to Complex1/1

== system bpsk_rx_coarse_sync/BPSK System/RF-DAC/NCO and Mixer/RF-DAC Coarse Mixer/fs_2 ==
  Data In : Inport
  Counter : dspswit3/Counter  Direction=Up  CountEvent=Free running  CounterSize=User defined  MaxCount=1  InitialCount=0  Output=Count  HitValue=32  ResetInput=off  SamplesPerFrame=ssr  Ts=1/(fs)  CntDtype=uint8  HitDtype=Logical
  Multiport Switch2 : MultiPortSwitch  DataPortOrder=Zero-based contiguous  Inputs=2  zeroidx=on
  Unary Minus : UnaryMinus
  Data Out : Outport  VectorParamsAs1DForOutWhenUnconnected=off
  wires:
  Data In/1 -> Unary Minus/1, Multiport Switch2/2
  Unary Minus/1 -> Multiport Switch2/3
  Counter/1 -> Multiport Switch2/1
  Multiport Switch2/1 -> Data Out/1

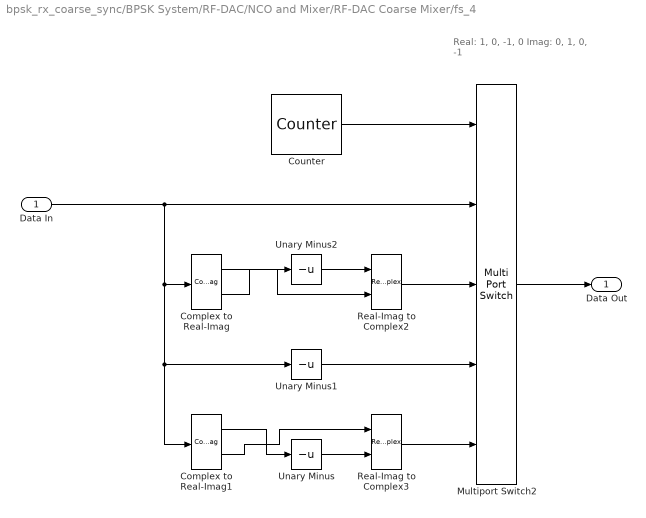
== system bpsk_rx_coarse_sync/BPSK System/RF-DAC/NCO and Mixer/RF-DAC Coarse Mixer/fs_4 ==
  note: Real:	1, 0, -1, 0
      | Imag:	0, 1, 0, -1
  Data In : Inport
  Complex to Real-Imag : ComplexToRealImag
  Complex to Real-Imag1 : ComplexToRealImag
  Counter : dspswit3/Counter  Direction=Up  CountEvent=Free running  CounterSize=User defined  MaxCount=3  InitialCount=0  Output=Count  HitValue=32  ResetInput=off  SamplesPerFrame=ssr  Ts=1/(fs)  CntDtype=uint8  HitDtype=Logical
  Multiport Switch2 : MultiPortSwitch  DataPortOrder=Zero-based contiguous  Inputs=4  zeroidx=on
  Real-Imag to Complex2 : RealImagToComplex
  Real-Imag to Complex3 : RealImagToComplex
  Unary Minus : UnaryMinus
  Unary Minus1 : UnaryMinus
  Unary Minus2 : UnaryMinus
  Data Out : Outport  VectorParamsAs1DForOutWhenUnconnected=off
  wires:
  Counter/1 -> Multiport Switch2/1
  Real-Imag to Complex2/1 -> Multiport Switch2/3
  Complex to Real-Imag/1 -> Real-Imag to Complex2/2
  Unary Minus1/1 -> Multiport Switch2/4
  Data In/1 -> Unary Minus1/1, Complex to Real-Imag1/1, Complex to Real-Imag/1, Multiport Switch2/2
  Real-Imag to Complex3/1 -> Multiport Switch2/5
  Multiport Switch2/1 -> Data Out/1
  Complex to Real-Imag1/2 -> Real-Imag to Complex3/1
  Complex to Real-Imag1/1 -> Unary Minus/1
  Unary Minus/1 -> Real-Imag to Complex3/2
  Complex to Real-Imag/2 -> Unary Minus2/1
  Unary Minus2/1 -> Real-Imag to Complex2/1
